simulink library "Controller_Bang_Bang"  (R2018b)
settings: Solver=ode45  StartTime=0.0  StopTime=10.0  RelTol=1e-3  EnableMultiTasking=on
settings Model: Creator=lena.frank  LastModifiedBy=P41573
settings DataIOCC: LimitDataPoints=on  SaveFormat=Array  SignalLoggingSaveFormat=ModelDataLogs
settings OptimizationCC: ExpressionDepthLimit=2147483647  LifeSpan=inf
settings DebuggingCC: UnderspecifiedInitializationDetection=Classic  MergeDetectMultiDrivingBlocksExec=none  SolverPrmCheckMsg=warning  FcnCallInpInsideContextMsg=warning  StateNameClashWarn=warning  SFUnexpectedBacktrackingDiag=warning  SFNoUnconditionalDefaultTransitionDiag=warning  SFExecutionAtInitializationDiag=none
settings HardwareCC: ProdBitPerPointer=32  ProdBitPerSizeT=32  ProdBitPerPtrDiffT=32  ProdLargestAtomicFloat=None  ProdIntDivRoundTo=Undefined  ProdEndianess=Unspecified  ProdWordSize=32  ProdHWDeviceType=32-bit Generic
settings ModelReferenceCC: PropagateSignalLabelsOutOfModel=off
settings SFSimCC: SimUseLocalCustomCode=off
settings RTWCC: RTWUseLocalCustomCode=off
settings CodeAppCC: StateflowObjectComments=on
settings GRTTargetCC: TargetLangStandard=C89/C90 (ANSI)  GeneratePreprocessorConditionals=Disable all  CombineOutputUpdateFcns=off  GRTInterface=on
settings ConfigComp: CovMetricSettings=dw  CovHtmlReporting=on  CovSaveCumulativeToWorkspaceVar=on  CovSaveSingleToWorkspaceVar=on  CovExternalEMLEnable=off

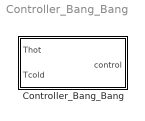
== system Controller_Bang_Bang ==
  Controller_Bang_Bang : Subsystem  mask(bang bang controler){deltaTon=5, deltaToff=1, Tmax=95}
      mask prompts: deltaTon "deltaT-on [K]"; deltaToff "deltaT-off [K]"; Tmax "maximum temperature [degree centigrade]"
      mask help:
      | Hysteresis controller for thermal systems. Output is set to zero if Thot or Tcold is bigger than Tmax.
      | deltaT = Thot - Tcold
      mask Help: web(fullfile(path_carnot('help'),'Controller_Bang_Bang.html'),'-helpbrowser')
      mask Display: plot(-30,0,150,100,[70,100,40,10,70,70,10,10],[50,80,80,50,50,20,20,50],[100,70],[50,20],[20,50,50,20,20],[40,40,30,30,40],[62,62,62,61,59,58,58,60],[42,41,39,38,38,40,42,43],[61,62,62,61,60,59,58,58,58,59],[32,31,30,28,27,28,28,30,31,32])

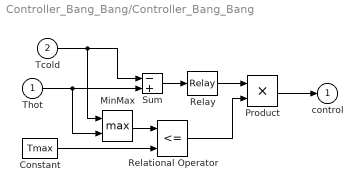
== system Controller_Bang_Bang/Controller_Bang_Bang ==
  Thot : Inport
  Tcold : Inport  Port=2
  Constant : Constant  Value=Tmax
  MinMax : MinMax  Function=max  Inputs=2  SaturateOnIntegerOverflow=on  InputSameDT=on
  Product : Product  OutDataTypeStr=double  SaturateOnIntegerOverflow=on
  Relational Operator : RelationalOperator  Operator=<=  RndMeth=Nearest  InputSameDT=on
  Relay : Relay  OnSwitchValue=deltaTon  OffSwitchValue=deltaToff
  Sum : Sum  Inputs=-+  SaturateOnIntegerOverflow=on  InputSameDT=on  OutDataTypeStr=Inherit: Same as first input
  control : Outport
  wires:
  Relational Operator/1 -> Product/2
  Product/1 -> control/1
  Relay/1 -> Product/1
  MinMax/1 -> Relational Operator/1
  Tcold/1 -> MinMax/1, Sum/1
  Thot/1 -> MinMax/2, Sum/2
  Constant/1 -> Relational Operator/2
  Sum/1 -> Relay/1
